simulink model "iff_sim"  (R2019b)
settings: Solver=VariableStepAuto  StartTime=0.0  StopTime=T  FixedStep=0.001  MaxStep=0.001  RelTol=1e-3
values from neighbouring files (symbols this model uses):
  bsc = 17    [model.mat]    (also in model_data.m)
  d_r = [0.01 0.01 0.01 0.01 0.01 0.01]    [model.mat]    (also in model_data.m = 0.01*ones(6,1))
  Fi_b_z = [0 2.09439510239 4.18879020479 1.0471975512 3.14159265359 5.23598775598]    [model.mat]    (also in model_data.m = [0;2/3;4/3;1/3;3/3;5/3]*pi)
  Fp = 148    [model.mat]    (also in model_data.m)
  ka = 11860000    [model.mat]    (also in model_data.m)
  Kd = 0    [ctc_data.m]
  Ki = 0    [ctc_data.m]
  Kp = 300    [ctc_data.m]
  ksc = 179000    [model.mat]    (also in model_data.m)
  l_r = [0.36 0.36 0.36 0.36 0.36 0.36]    [model.mat]    (also in model_data.m = 0.36*ones(6,1))
  la00 = 0.061    [model.mat]    (also in model_data.m)
  O_lb = [0 0 0 0 0 0]    [model.mat]    (also in model_data.m = [0;0;0;0;0;0])
  q_d = out_ik.q'    [ik_run.m]
  qt_d = out_ik.qt'    [ik_run.m]
  qtt_d = out_ik.qtt'    [ik_run.m]
  RMSforce = 35    [model.mat]
  s = out_ctc.s    [ctc_run.m]
  s_0 = s_d(:,:,1)    [ctc_run.m]    (also in iff_run.m)
  T = 1.5    [ctc_data.m]
  t_d = out_ik.t'    [ik_run.m]
  t_dist = 0.1    [model.mat]
  ts_noise = 1.6e-05    [model.mat]    (also in model_data.m)
  v_0 = v_d(:,:,1)    [ctc_run.m]    (also in iff_run.m)
  w_lb = 0.195    [model.mat]    (also in model_data.m)
  W_lb = 0.205    [model.mat]    (also in model_data.m)
  w_ub = 0.195    [model.mat]    (also in model_data.m)
  W_ub = 0.205    [model.mat]    (also in model_data.m)
undefined symbols (not defined in the file or in its folder): X, Y, Z
libraries: nesl_utility x282, sm_lib x208, dspindex x30, simulink x12, powerlib_meascontrol x1
(part 13 of 14)

== system iff_sim/High-authority control/CTC/computed torque control/desired cable vectors// lengths/cable 8 ==
  Cylindrical Joint : sm_lib/Joints/Cylindrical Joint  JointMode=Normal  SenseConstraintForce=off  SenseConstraintForceX=off  SenseConstraintForceY=off  SenseConstraintForceZ=off  SenseConstraintTorque=off  SenseConstraintTorqueX=off  SenseConstraintTorqueY=off  SenseConstraintTorqueZ=off  SenseTotalForce=off  SenseTotalForceX=off  SenseTotalForceY=off  SenseTotalForceZ=off  SenseTotalTorque=off  SenseTotalTorqueX=off  SenseTotalTorqueY=off  SenseTotalTorqueZ=off  CompositeWrenchDir=FollowerOnBase  CompositeWrenchFrame=BaseFrame  PzEquilibriumPosition=0  PzEquilibriumPositionUnits=m  PzSpringStiffness=0  PzSpringStiffnessUnits=N/m  PzDampingCoefficient=0  PzDampingCoefficientUnits=N/(m/s)  PzTorqueActuationMode=ComputedTorque  PzMotionActuationMode=ComputedMotion  PzSensePosition=on  PzSenseVelocity=off  PzSenseAcceleration=off  PzSenseTorqueForce=on  PzSenseLowerLimitTorqueForce=off  PzSenseUpperLimitTorqueForce=off  PzLowerLimitSpecify=off  PzLowerLimitBound=-1  PzLowerLimitBoundUnits=m  PzLowerLimitStiffness=1e6  PzLowerLimitStiffnessUnits=N/m  PzLowerLimitDamping=1e3  PzLowerLimitDampingUnits=N/(m/s)  PzLowerLimitTransitionRegionWidth=1e-4  PzLowerLimitTransitionRegionWidthUnits=m  PzUpperLimitSpecify=off  PzUpperLimitBound=1  PzUpperLimitBoundUnits=m  PzUpperLimitStiffness=1e6  PzUpperLimitStiffnessUnits=N/m  PzUpperLimitDamping=1e3  PzUpperLimitDampingUnits=N/(m/s)  PzUpperLimitTransitionRegionWidth=1e-4  PzUpperLimitTransitionRegionWidthUnits=m  PzPositionTargetSpecify=on  PzPositionTargetPriority=Low  PzPositionTargetValue=1  PzPositionTargetValueUnits=m  PzVelocityTargetSpecify=off  PzVelocityTargetPriority=High  PzVelocityTargetValue=0  PzVelocityTargetValueUnits=m/s  RzEquilibriumPosition=0  RzEquilibriumPositionUnits=deg  RzSpringStiffness=0  RzSpringStiffnessUnits=N*m/deg  RzDampingCoefficient=0  RzDampingCoefficientUnits=N*m/(deg/s)  RzTorqueActuationMode=NoTorque  RzMotionActuationMode=ComputedMotion  RzSensePosition=off  RzSenseVelocity=off  RzSenseAcceleration=off  RzSenseTorqueForce=off  RzSenseLowerLimitTorqueForce=off  RzSenseUpperLimitTorqueForce=off  RzLowerLimitSpecify=off  RzLowerLimitBound=-90  RzLowerLimitBoundUnits=deg  RzLowerLimitStiffness=1e4  RzLowerLimitStiffnessUnits=N*m/deg  RzLowerLimitDamping=10  RzLowerLimitDampingUnits=N*m/(deg/s)  RzLowerLimitTransitionRegionWidth=0.1  RzLowerLimitTransitionRegionWidthUnits=deg  RzUpperLimitSpecify=off  RzUpperLimitBound=90  RzUpperLimitBoundUnits=deg  RzUpperLimitStiffness=1e4  RzUpperLimitStiffnessUnits=N*m/deg  RzUpperLimitDamping=10  RzUpperLimitDampingUnits=N*m/(deg/s)  RzUpperLimitTransitionRegionWidth=0.1  RzUpperLimitTransitionRegionWidthUnits=deg  RzPositionTargetSpecify=off  RzPositionTargetPriority=High  RzPositionTargetValue=0  RzPositionTargetValueUnits=deg  RzVelocityTargetSpecify=off  RzVelocityTargetPriority=High  RzVelocityTargetValue=0  RzVelocityTargetValueUnits=deg/s
  PS-Simulink Converter : nesl_utility/PS-Simulink Converter  PhysicalDomain=network_engine_domain  SubClassName=ps_output  LeftPortType=input  RightPortType=output  PseudoPeriodic=off  Frequencies=[]  Unit=m  AffineConversion=off
  PS-Simulink Converter1 : nesl_utility/PS-Simulink Converter  PhysicalDomain=network_engine_domain  SubClassName=ps_output  LeftPortType=input  RightPortType=output  PseudoPeriodic=off  Frequencies=[]  Unit=N  AffineConversion=off
  Universal Joint : sm_lib/Joints/Universal Joint  JointMode=Normal  SenseConstraintForce=off  SenseConstraintForceX=off  SenseConstraintForceY=off  SenseConstraintForceZ=off  SenseConstraintTorque=off  SenseConstraintTorqueX=off  SenseConstraintTorqueY=off  SenseConstraintTorqueZ=off  SenseTotalForce=off  SenseTotalForceX=off  SenseTotalForceY=off  SenseTotalForceZ=off  SenseTotalTorque=off  SenseTotalTorqueX=off  SenseTotalTorqueY=off  SenseTotalTorqueZ=off  CompositeWrenchDir=FollowerOnBase  CompositeWrenchFrame=BaseFrame  RxEquilibriumPosition=0  RxEquilibriumPositionUnits=deg  RxSpringStiffness=0  RxSpringStiffnessUnits=N*m/deg  RxDampingCoefficient=0  RxDampingCoefficientUnits=N*m/(deg/s)  RxTorqueActuationMode=NoTorque  RxMotionActuationMode=ComputedMotion  RxSensePosition=off  RxSenseVelocity=off  RxSenseAcceleration=off  RxSenseTorqueForce=off  RxSenseLowerLimitTorqueForce=off  RxSenseUpperLimitTorqueForce=off  RxLowerLimitSpecify=off  RxLowerLimitBound=-90  RxLowerLimitBoundUnits=deg  RxLowerLimitStiffness=1e4  RxLowerLimitStiffnessUnits=N*m/deg  RxLowerLimitDamping=10  RxLowerLimitDampingUnits=N*m/(deg/s)  RxLowerLimitTransitionRegionWidth=0.1  RxLowerLimitTransitionRegionWidthUnits=deg  RxUpperLimitSpecify=off  RxUpperLimitBound=90  RxUpperLimitBoundUnits=deg  RxUpperLimitStiffness=1e4  RxUpperLimitStiffnessUnits=N*m/deg  RxUpperLimitDamping=10  RxUpperLimitDampingUnits=N*m/(deg/s)  RxUpperLimitTransitionRegionWidth=0.1  RxUpperLimitTransitionRegionWidthUnits=deg  RxPositionTargetSpecify=off  RxPositionTargetPriority=High  RxPositionTargetValue=0  RxPositionTargetValueUnits=deg  RxVelocityTargetSpecify=off  RxVelocityTargetPriority=High  RxVelocityTargetValue=0  RxVelocityTargetValueUnits=deg/s  RyEquilibriumPosition=0  RyEquilibriumPositionUnits=deg  RySpringStiffness=0  RySpringStiffnessUnits=N*m/deg  RyDampingCoefficient=0  RyDampingCoefficientUnits=N*m/(deg/s)  RyTorqueActuationMode=NoTorque  RyMotionActuationMode=ComputedMotion  RySensePosition=off  RySenseVelocity=off  RySenseAcceleration=off  RySenseTorqueForce=off  RySenseLowerLimitTorqueForce=off  RySenseUpperLimitTorqueForce=off  RyLowerLimitSpecify=off  RyLowerLimitBound=-90  RyLowerLimitBoundUnits=deg  RyLowerLimitStiffness=1e4  RyLowerLimitStiffnessUnits=N*m/deg  RyLowerLimitDamping=10  RyLowerLimitDampingUnits=N*m/(deg/s)  RyLowerLimitTransitionRegionWidth=0.1  RyLowerLimitTransitionRegionWidthUnits=deg  RyUpperLimitSpecify=off  RyUpperLimitBound=90  RyUpperLimitBoundUnits=deg  RyUpperLimitStiffness=1e4  RyUpperLimitStiffnessUnits=N*m/deg  RyUpperLimitDamping=10  RyUpperLimitDampingUnits=N*m/(deg/s)  RyUpperLimitTransitionRegionWidth=0.1  RyUpperLimitTransitionRegionWidthUnits=deg  RyPositionTargetSpecify=off  RyPositionTargetPriority=High  RyPositionTargetValue=0  RyPositionTargetValueUnits=deg  RyVelocityTargetSpecify=off  RyVelocityTargetPriority=High  RyVelocityTargetValue=0  RyVelocityTargetValueUnits=deg/s
      settings: SourceProductName=Simscape Multibody
  Universal Joint1 : sm_lib/Joints/Universal Joint  JointMode=Normal  SenseConstraintForce=off  SenseConstraintForceX=off  SenseConstraintForceY=off  SenseConstraintForceZ=off  SenseConstraintTorque=off  SenseConstraintTorqueX=off  SenseConstraintTorqueY=off  SenseConstraintTorqueZ=off  SenseTotalForce=off  SenseTotalForceX=off  SenseTotalForceY=off  SenseTotalForceZ=off  SenseTotalTorque=off  SenseTotalTorqueX=off  SenseTotalTorqueY=off  SenseTotalTorqueZ=off  CompositeWrenchDir=FollowerOnBase  CompositeWrenchFrame=BaseFrame  RxEquilibriumPosition=0  RxEquilibriumPositionUnits=deg  RxSpringStiffness=0  RxSpringStiffnessUnits=N*m/deg  RxDampingCoefficient=0  RxDampingCoefficientUnits=N*m/(deg/s)  RxTorqueActuationMode=NoTorque  RxMotionActuationMode=ComputedMotion  RxSensePosition=off  RxSenseVelocity=off  RxSenseAcceleration=off  RxSenseTorqueForce=off  RxSenseLowerLimitTorqueForce=off  RxSenseUpperLimitTorqueForce=off  RxLowerLimitSpecify=off  RxLowerLimitBound=-90  RxLowerLimitBoundUnits=deg  RxLowerLimitStiffness=1e4  RxLowerLimitStiffnessUnits=N*m/deg  RxLowerLimitDamping=10  RxLowerLimitDampingUnits=N*m/(deg/s)  RxLowerLimitTransitionRegionWidth=0.1  RxLowerLimitTransitionRegionWidthUnits=deg  RxUpperLimitSpecify=off  RxUpperLimitBound=90  RxUpperLimitBoundUnits=deg  RxUpperLimitStiffness=1e4  RxUpperLimitStiffnessUnits=N*m/deg  RxUpperLimitDamping=10  RxUpperLimitDampingUnits=N*m/(deg/s)  RxUpperLimitTransitionRegionWidth=0.1  RxUpperLimitTransitionRegionWidthUnits=deg  RxPositionTargetSpecify=off  RxPositionTargetPriority=High  RxPositionTargetValue=0  RxPositionTargetValueUnits=deg  RxVelocityTargetSpecify=off  RxVelocityTargetPriority=High  RxVelocityTargetValue=0  RxVelocityTargetValueUnits=deg/s  RyEquilibriumPosition=0  RyEquilibriumPositionUnits=deg  RySpringStiffness=0  RySpringStiffnessUnits=N*m/deg  RyDampingCoefficient=0  RyDampingCoefficientUnits=N*m/(deg/s)  RyTorqueActuationMode=NoTorque  RyMotionActuationMode=ComputedMotion  RySensePosition=off  RySenseVelocity=off  RySenseAcceleration=off  RySenseTorqueForce=off  RySenseLowerLimitTorqueForce=off  RySenseUpperLimitTorqueForce=off  RyLowerLimitSpecify=off  RyLowerLimitBound=-90  RyLowerLimitBoundUnits=deg  RyLowerLimitStiffness=1e4  RyLowerLimitStiffnessUnits=N*m/deg  RyLowerLimitDamping=10  RyLowerLimitDampingUnits=N*m/(deg/s)  RyLowerLimitTransitionRegionWidth=0.1  RyLowerLimitTransitionRegionWidthUnits=deg  RyUpperLimitSpecify=off  RyUpperLimitBound=90  RyUpperLimitBoundUnits=deg  RyUpperLimitStiffness=1e4  RyUpperLimitStiffnessUnits=N*m/deg  RyUpperLimitDamping=10  RyUpperLimitDampingUnits=N*m/(deg/s)  RyUpperLimitTransitionRegionWidth=0.1  RyUpperLimitTransitionRegionWidthUnits=deg  RyPositionTargetSpecify=off  RyPositionTargetPriority=High  RyPositionTargetValue=0  RyPositionTargetValueUnits=deg  RyVelocityTargetSpecify=off  RyVelocityTargetPriority=High  RyVelocityTargetValue=0  RyVelocityTargetValueUnits=deg/s
      settings: SourceProductName=Simscape Multibody
  cable force and length : MATLAB Function  TreatAsAtomicUnit=on
  K_c : PMIOPort  Side=Left
  L_c : PMIOPort  Port=2  Side=Right
  F_c : Outport
  l_c : Outport  Port=2
  wires:
  PS-Simulink Converter/1 -> cable force and length/1(pz)
  PS-Simulink Converter1/1 -> cable force and length/2(fz)
  cable force and length/1(F_c) -> F_c/1
  cable force and length/2(l_c) -> l_c/1
  connections:
  Universal Joint/LConn1 -- K_c/RConn1
  Cylindrical Joint/LConn1 -- Universal Joint/RConn1
  L_c/RConn1 -- Universal Joint1/RConn1
  Universal Joint1/LConn1 -- Cylindrical Joint/RConn1
  PS-Simulink Converter/LConn1 -- Cylindrical Joint/RConn2
  PS-Simulink Converter1/LConn1 -- Cylindrical Joint/RConn3

== system iff_sim/High-authority control/CTC/computed torque control/desired cable vectors// lengths/cable 9 ==
  Cylindrical Joint : sm_lib/Joints/Cylindrical Joint  JointMode=Normal  SenseConstraintForce=off  SenseConstraintForceX=off  SenseConstraintForceY=off  SenseConstraintForceZ=off  SenseConstraintTorque=off  SenseConstraintTorqueX=off  SenseConstraintTorqueY=off  SenseConstraintTorqueZ=off  SenseTotalForce=off  SenseTotalForceX=off  SenseTotalForceY=off  SenseTotalForceZ=off  SenseTotalTorque=off  SenseTotalTorqueX=off  SenseTotalTorqueY=off  SenseTotalTorqueZ=off  CompositeWrenchDir=FollowerOnBase  CompositeWrenchFrame=BaseFrame  PzEquilibriumPosition=0  PzEquilibriumPositionUnits=m  PzSpringStiffness=0  PzSpringStiffnessUnits=N/m  PzDampingCoefficient=0  PzDampingCoefficientUnits=N/(m/s)  PzTorqueActuationMode=ComputedTorque  PzMotionActuationMode=ComputedMotion  PzSensePosition=on  PzSenseVelocity=off  PzSenseAcceleration=off  PzSenseTorqueForce=on  PzSenseLowerLimitTorqueForce=off  PzSenseUpperLimitTorqueForce=off  PzLowerLimitSpecify=off  PzLowerLimitBound=-1  PzLowerLimitBoundUnits=m  PzLowerLimitStiffness=1e6  PzLowerLimitStiffnessUnits=N/m  PzLowerLimitDamping=1e3  PzLowerLimitDampingUnits=N/(m/s)  PzLowerLimitTransitionRegionWidth=1e-4  PzLowerLimitTransitionRegionWidthUnits=m  PzUpperLimitSpecify=off  PzUpperLimitBound=1  PzUpperLimitBoundUnits=m  PzUpperLimitStiffness=1e6  PzUpperLimitStiffnessUnits=N/m  PzUpperLimitDamping=1e3  PzUpperLimitDampingUnits=N/(m/s)  PzUpperLimitTransitionRegionWidth=1e-4  PzUpperLimitTransitionRegionWidthUnits=m  PzPositionTargetSpecify=on  PzPositionTargetPriority=Low  PzPositionTargetValue=1  PzPositionTargetValueUnits=m  PzVelocityTargetSpecify=off  PzVelocityTargetPriority=High  PzVelocityTargetValue=0  PzVelocityTargetValueUnits=m/s  RzEquilibriumPosition=0  RzEquilibriumPositionUnits=deg  RzSpringStiffness=0  RzSpringStiffnessUnits=N*m/deg  RzDampingCoefficient=0  RzDampingCoefficientUnits=N*m/(deg/s)  RzTorqueActuationMode=NoTorque  RzMotionActuationMode=ComputedMotion  RzSensePosition=off  RzSenseVelocity=off  RzSenseAcceleration=off  RzSenseTorqueForce=off  RzSenseLowerLimitTorqueForce=off  RzSenseUpperLimitTorqueForce=off  RzLowerLimitSpecify=off  RzLowerLimitBound=-90  RzLowerLimitBoundUnits=deg  RzLowerLimitStiffness=1e4  RzLowerLimitStiffnessUnits=N*m/deg  RzLowerLimitDamping=10  RzLowerLimitDampingUnits=N*m/(deg/s)  RzLowerLimitTransitionRegionWidth=0.1  RzLowerLimitTransitionRegionWidthUnits=deg  RzUpperLimitSpecify=off  RzUpperLimitBound=90  RzUpperLimitBoundUnits=deg  RzUpperLimitStiffness=1e4  RzUpperLimitStiffnessUnits=N*m/deg  RzUpperLimitDamping=10  RzUpperLimitDampingUnits=N*m/(deg/s)  RzUpperLimitTransitionRegionWidth=0.1  RzUpperLimitTransitionRegionWidthUnits=deg  RzPositionTargetSpecify=off  RzPositionTargetPriority=High  RzPositionTargetValue=0  RzPositionTargetValueUnits=deg  RzVelocityTargetSpecify=off  RzVelocityTargetPriority=High  RzVelocityTargetValue=0  RzVelocityTargetValueUnits=deg/s
  PS-Simulink Converter : nesl_utility/PS-Simulink Converter  PhysicalDomain=network_engine_domain  SubClassName=ps_output  LeftPortType=input  RightPortType=output  PseudoPeriodic=off  Frequencies=[]  Unit=m  AffineConversion=off
  PS-Simulink Converter1 : nesl_utility/PS-Simulink Converter  PhysicalDomain=network_engine_domain  SubClassName=ps_output  LeftPortType=input  RightPortType=output  PseudoPeriodic=off  Frequencies=[]  Unit=N  AffineConversion=off
  Universal Joint : sm_lib/Joints/Universal Joint  JointMode=Normal  SenseConstraintForce=off  SenseConstraintForceX=off  SenseConstraintForceY=off  SenseConstraintForceZ=off  SenseConstraintTorque=off  SenseConstraintTorqueX=off  SenseConstraintTorqueY=off  SenseConstraintTorqueZ=off  SenseTotalForce=off  SenseTotalForceX=off  SenseTotalForceY=off  SenseTotalForceZ=off  SenseTotalTorque=off  SenseTotalTorqueX=off  SenseTotalTorqueY=off  SenseTotalTorqueZ=off  CompositeWrenchDir=FollowerOnBase  CompositeWrenchFrame=BaseFrame  RxEquilibriumPosition=0  RxEquilibriumPositionUnits=deg  RxSpringStiffness=0  RxSpringStiffnessUnits=N*m/deg  RxDampingCoefficient=0  RxDampingCoefficientUnits=N*m/(deg/s)  RxTorqueActuationMode=NoTorque  RxMotionActuationMode=ComputedMotion  RxSensePosition=off  RxSenseVelocity=off  RxSenseAcceleration=off  RxSenseTorqueForce=off  RxSenseLowerLimitTorqueForce=off  RxSenseUpperLimitTorqueForce=off  RxLowerLimitSpecify=off  RxLowerLimitBound=-90  RxLowerLimitBoundUnits=deg  RxLowerLimitStiffness=1e4  RxLowerLimitStiffnessUnits=N*m/deg  RxLowerLimitDamping=10  RxLowerLimitDampingUnits=N*m/(deg/s)  RxLowerLimitTransitionRegionWidth=0.1  RxLowerLimitTransitionRegionWidthUnits=deg  RxUpperLimitSpecify=off  RxUpperLimitBound=90  RxUpperLimitBoundUnits=deg  RxUpperLimitStiffness=1e4  RxUpperLimitStiffnessUnits=N*m/deg  RxUpperLimitDamping=10  RxUpperLimitDampingUnits=N*m/(deg/s)  RxUpperLimitTransitionRegionWidth=0.1  RxUpperLimitTransitionRegionWidthUnits=deg  RxPositionTargetSpecify=off  RxPositionTargetPriority=High  RxPositionTargetValue=0  RxPositionTargetValueUnits=deg  RxVelocityTargetSpecify=off  RxVelocityTargetPriority=High  RxVelocityTargetValue=0  RxVelocityTargetValueUnits=deg/s  RyEquilibriumPosition=0  RyEquilibriumPositionUnits=deg  RySpringStiffness=0  RySpringStiffnessUnits=N*m/deg  RyDampingCoefficient=0  RyDampingCoefficientUnits=N*m/(deg/s)  RyTorqueActuationMode=NoTorque  RyMotionActuationMode=ComputedMotion  RySensePosition=off  RySenseVelocity=off  RySenseAcceleration=off  RySenseTorqueForce=off  RySenseLowerLimitTorqueForce=off  RySenseUpperLimitTorqueForce=off  RyLowerLimitSpecify=off  RyLowerLimitBound=-90  RyLowerLimitBoundUnits=deg  RyLowerLimitStiffness=1e4  RyLowerLimitStiffnessUnits=N*m/deg  RyLowerLimitDamping=10  RyLowerLimitDampingUnits=N*m/(deg/s)  RyLowerLimitTransitionRegionWidth=0.1  RyLowerLimitTransitionRegionWidthUnits=deg  RyUpperLimitSpecify=off  RyUpperLimitBound=90  RyUpperLimitBoundUnits=deg  RyUpperLimitStiffness=1e4  RyUpperLimitStiffnessUnits=N*m/deg  RyUpperLimitDamping=10  RyUpperLimitDampingUnits=N*m/(deg/s)  RyUpperLimitTransitionRegionWidth=0.1  RyUpperLimitTransitionRegionWidthUnits=deg  RyPositionTargetSpecify=off  RyPositionTargetPriority=High  RyPositionTargetValue=0  RyPositionTargetValueUnits=deg  RyVelocityTargetSpecify=off  RyVelocityTargetPriority=High  RyVelocityTargetValue=0  RyVelocityTargetValueUnits=deg/s
      settings: SourceProductName=Simscape Multibody
  Universal Joint1 : sm_lib/Joints/Universal Joint  JointMode=Normal  SenseConstraintForce=off  SenseConstraintForceX=off  SenseConstraintForceY=off  SenseConstraintForceZ=off  SenseConstraintTorque=off  SenseConstraintTorqueX=off  SenseConstraintTorqueY=off  SenseConstraintTorqueZ=off  SenseTotalForce=off  SenseTotalForceX=off  SenseTotalForceY=off  SenseTotalForceZ=off  SenseTotalTorque=off  SenseTotalTorqueX=off  SenseTotalTorqueY=off  SenseTotalTorqueZ=off  CompositeWrenchDir=FollowerOnBase  CompositeWrenchFrame=BaseFrame  RxEquilibriumPosition=0  RxEquilibriumPositionUnits=deg  RxSpringStiffness=0  RxSpringStiffnessUnits=N*m/deg  RxDampingCoefficient=0  RxDampingCoefficientUnits=N*m/(deg/s)  RxTorqueActuationMode=NoTorque  RxMotionActuationMode=ComputedMotion  RxSensePosition=off  RxSenseVelocity=off  RxSenseAcceleration=off  RxSenseTorqueForce=off  RxSenseLowerLimitTorqueForce=off  RxSenseUpperLimitTorqueForce=off  RxLowerLimitSpecify=off  RxLowerLimitBound=-90  RxLowerLimitBoundUnits=deg  RxLowerLimitStiffness=1e4  RxLowerLimitStiffnessUnits=N*m/deg  RxLowerLimitDamping=10  RxLowerLimitDampingUnits=N*m/(deg/s)  RxLowerLimitTransitionRegionWidth=0.1  RxLowerLimitTransitionRegionWidthUnits=deg  RxUpperLimitSpecify=off  RxUpperLimitBound=90  RxUpperLimitBoundUnits=deg  RxUpperLimitStiffness=1e4  RxUpperLimitStiffnessUnits=N*m/deg  RxUpperLimitDamping=10  RxUpperLimitDampingUnits=N*m/(deg/s)  RxUpperLimitTransitionRegionWidth=0.1  RxUpperLimitTransitionRegionWidthUnits=deg  RxPositionTargetSpecify=off  RxPositionTargetPriority=High  RxPositionTargetValue=0  RxPositionTargetValueUnits=deg  RxVelocityTargetSpecify=off  RxVelocityTargetPriority=High  RxVelocityTargetValue=0  RxVelocityTargetValueUnits=deg/s  RyEquilibriumPosition=0  RyEquilibriumPositionUnits=deg  RySpringStiffness=0  RySpringStiffnessUnits=N*m/deg  RyDampingCoefficient=0  RyDampingCoefficientUnits=N*m/(deg/s)  RyTorqueActuationMode=NoTorque  RyMotionActuationMode=ComputedMotion  RySensePosition=off  RySenseVelocity=off  RySenseAcceleration=off  RySenseTorqueForce=off  RySenseLowerLimitTorqueForce=off  RySenseUpperLimitTorqueForce=off  RyLowerLimitSpecify=off  RyLowerLimitBound=-90  RyLowerLimitBoundUnits=deg  RyLowerLimitStiffness=1e4  RyLowerLimitStiffnessUnits=N*m/deg  RyLowerLimitDamping=10  RyLowerLimitDampingUnits=N*m/(deg/s)  RyLowerLimitTransitionRegionWidth=0.1  RyLowerLimitTransitionRegionWidthUnits=deg  RyUpperLimitSpecify=off  RyUpperLimitBound=90  RyUpperLimitBoundUnits=deg  RyUpperLimitStiffness=1e4  RyUpperLimitStiffnessUnits=N*m/deg  RyUpperLimitDamping=10  RyUpperLimitDampingUnits=N*m/(deg/s)  RyUpperLimitTransitionRegionWidth=0.1  RyUpperLimitTransitionRegionWidthUnits=deg  RyPositionTargetSpecify=off  RyPositionTargetPriority=High  RyPositionTargetValue=0  RyPositionTargetValueUnits=deg  RyVelocityTargetSpecify=off  RyVelocityTargetPriority=High  RyVelocityTargetValue=0  RyVelocityTargetValueUnits=deg/s
      settings: SourceProductName=Simscape Multibody
  cable force and length : MATLAB Function  TreatAsAtomicUnit=on
  K_c : PMIOPort  Side=Left
  L_c : PMIOPort  Port=2  Side=Right
  F_c : Outport
  l_c : Outport  Port=2
  wires:
  PS-Simulink Converter/1 -> cable force and length/1(pz)
  PS-Simulink Converter1/1 -> cable force and length/2(fz)
  cable force and length/1(F_c) -> F_c/1
  cable force and length/2(l_c) -> l_c/1
  connections:
  Universal Joint/LConn1 -- K_c/RConn1
  Cylindrical Joint/LConn1 -- Universal Joint/RConn1
  L_c/RConn1 -- Universal Joint1/RConn1
  Universal Joint1/LConn1 -- Cylindrical Joint/RConn1
  PS-Simulink Converter/LConn1 -- Cylindrical Joint/RConn2
  PS-Simulink Converter1/LConn1 -- Cylindrical Joint/RConn3

== system iff_sim/High-authority control/CTC/inverse kinematics/t -> q_d/rod 1 ==
  t : Inport
  Mux : Mux  Inputs=2
  Q_r,d,x : Lookup_n-D  NumberOfTableDimensions=1  BreakpointsForDimension1=t_d(1,:)  BreakpointsForDimension2=t_d(1,:)  Table=Q_d((r-1)*2+1,:)  InternalRulePriority=Speed  RndMeth=Simplest  InputSameDT=on
  Q_r,d,y : Lookup_n-D  NumberOfTableDimensions=1  BreakpointsForDimension1=t_d(1,:)  BreakpointsForDimension2=t_d(1,:)  Table=Q_d((r-1)*2+2,:)  InternalRulePriority=Speed  RndMeth=Simplest  InputSameDT=on
  Q_r,d : Outport
  wires:
  t/1 -> Q_r,d,y/1, Q_r,d,x/1
  Q_r,d,y/1 -> Mux/2
  Q_r,d,x/1 -> Mux/1
  Mux/1 -> Q_r,d/1

== system iff_sim/High-authority control/CTC/inverse kinematics/t -> q_d/rod 2 ==
  t : Inport
  Mux : Mux  Inputs=2
  Q_r,d,x : Lookup_n-D  NumberOfTableDimensions=1  BreakpointsForDimension1=t_d(1,:)  BreakpointsForDimension2=t_d(1,:)  Table=Q_d((r-1)*2+1,:)  InternalRulePriority=Speed  RndMeth=Simplest  InputSameDT=on
  Q_r,d,y : Lookup_n-D  NumberOfTableDimensions=1  BreakpointsForDimension1=t_d(1,:)  BreakpointsForDimension2=t_d(1,:)  Table=Q_d((r-1)*2+2,:)  InternalRulePriority=Speed  RndMeth=Simplest  InputSameDT=on
  Q_r,d : Outport
  wires:
  t/1 -> Q_r,d,y/1, Q_r,d,x/1
  Q_r,d,y/1 -> Mux/2
  Q_r,d,x/1 -> Mux/1
  Mux/1 -> Q_r,d/1

== system iff_sim/High-authority control/CTC/inverse kinematics/t -> q_d/rod 3 ==
  t : Inport
  Mux : Mux  Inputs=2
  Q_r,d,x : Lookup_n-D  NumberOfTableDimensions=1  BreakpointsForDimension1=t_d(1,:)  BreakpointsForDimension2=t_d(1,:)  Table=Q_d((r-1)*2+1,:)  InternalRulePriority=Speed  RndMeth=Simplest  InputSameDT=on
  Q_r,d,y : Lookup_n-D  NumberOfTableDimensions=1  BreakpointsForDimension1=t_d(1,:)  BreakpointsForDimension2=t_d(1,:)  Table=Q_d((r-1)*2+2,:)  InternalRulePriority=Speed  RndMeth=Simplest  InputSameDT=on
  Q_r,d : Outport
  wires:
  t/1 -> Q_r,d,y/1, Q_r,d,x/1
  Q_r,d,y/1 -> Mux/2
  Q_r,d,x/1 -> Mux/1
  Mux/1 -> Q_r,d/1

== system iff_sim/High-authority control/CTC/inverse kinematics/t -> q_d/rod 4 ==
  t : Inport
  Mux : Mux  Inputs=2
  Q_r,d,x : Lookup_n-D  NumberOfTableDimensions=1  BreakpointsForDimension1=t_d(1,:)  BreakpointsForDimension2=t_d(1,:)  Table=Q_d((r-1)*2+1,:)  InternalRulePriority=Speed  RndMeth=Simplest  InputSameDT=on
  Q_r,d,y : Lookup_n-D  NumberOfTableDimensions=1  BreakpointsForDimension1=t_d(1,:)  BreakpointsForDimension2=t_d(1,:)  Table=Q_d((r-1)*2+2,:)  InternalRulePriority=Speed  RndMeth=Simplest  InputSameDT=on
  Q_r,d : Outport
  wires:
  t/1 -> Q_r,d,y/1, Q_r,d,x/1
  Q_r,d,y/1 -> Mux/2
  Q_r,d,x/1 -> Mux/1
  Mux/1 -> Q_r,d/1

== system iff_sim/High-authority control/CTC/inverse kinematics/t -> q_d/rod 5 ==
  t : Inport
  Mux : Mux  Inputs=2
  Q_r,d,x : Lookup_n-D  NumberOfTableDimensions=1  BreakpointsForDimension1=t_d(1,:)  BreakpointsForDimension2=t_d(1,:)  Table=Q_d((r-1)*2+1,:)  InternalRulePriority=Speed  RndMeth=Simplest  InputSameDT=on
  Q_r,d,y : Lookup_n-D  NumberOfTableDimensions=1  BreakpointsForDimension1=t_d(1,:)  BreakpointsForDimension2=t_d(1,:)  Table=Q_d((r-1)*2+2,:)  InternalRulePriority=Speed  RndMeth=Simplest  InputSameDT=on
  Q_r,d : Outport
  wires:
  t/1 -> Q_r,d,y/1, Q_r,d,x/1
  Q_r,d,y/1 -> Mux/2
  Q_r,d,x/1 -> Mux/1
  Mux/1 -> Q_r,d/1

== system iff_sim/High-authority control/CTC/inverse kinematics/t -> q_d/rod 6 ==
  t : Inport
  Mux : Mux  Inputs=2
  Q_r,d,x : Lookup_n-D  NumberOfTableDimensions=1  BreakpointsForDimension1=t_d(1,:)  BreakpointsForDimension2=t_d(1,:)  Table=Q_d((r-1)*2+1,:)  InternalRulePriority=Speed  RndMeth=Simplest  InputSameDT=on
  Q_r,d,y : Lookup_n-D  NumberOfTableDimensions=1  BreakpointsForDimension1=t_d(1,:)  BreakpointsForDimension2=t_d(1,:)  Table=Q_d((r-1)*2+2,:)  InternalRulePriority=Speed  RndMeth=Simplest  InputSameDT=on
  Q_r,d : Outport
  wires:
  t/1 -> Q_r,d,y/1, Q_r,d,x/1
  Q_r,d,y/1 -> Mux/2
  Q_r,d,x/1 -> Mux/1
  Mux/1 -> Q_r,d/1

== system iff_sim/High-authority control/CTC/inverse kinematics/t -> q_d/upper base ==
  t : Inport
  Mux : Mux  Inputs=6
  Q_ub,d,phi_x : Lookup_n-D  NumberOfTableDimensions=1  BreakpointsForDimension1=t_d(1,:)  BreakpointsForDimension2=t_d(1,:)  Table=Q_d(16,:)  InternalRulePriority=Speed  RndMeth=Simplest  InputSameDT=on
  Q_ub,d,phi_y : Lookup_n-D  NumberOfTableDimensions=1  BreakpointsForDimension1=t_d(1,:)  BreakpointsForDimension2=t_d(1,:)  Table=Q_d(17,:)  InternalRulePriority=Speed  RndMeth=Simplest  InputSameDT=on
  Q_ub,d,phi_z : Lookup_n-D  NumberOfTableDimensions=1  BreakpointsForDimension1=t_d(1,:)  BreakpointsForDimension2=t_d(1,:)  Table=Q_d(18,:)  InternalRulePriority=Speed  RndMeth=Simplest  InputSameDT=on
  Q_ub,d,x : Lookup_n-D  NumberOfTableDimensions=1  BreakpointsForDimension1=t_d(1,:)  BreakpointsForDimension2=t_d(1,:)  Table=Q_d(13,:)  InternalRulePriority=Speed  RndMeth=Simplest  InputSameDT=on
  Q_ub,d,y : Lookup_n-D  NumberOfTableDimensions=1  BreakpointsForDimension1=t_d(1,:)  BreakpointsForDimension2=t_d(1,:)  Table=Q_d(14,:)  InternalRulePriority=Speed  RndMeth=Simplest  InputSameDT=on
  Q_ub,d,z : Lookup_n-D  NumberOfTableDimensions=1  BreakpointsForDimension1=t_d(1,:)  BreakpointsForDimension2=t_d(1,:)  Table=Q_d(15,:)  InternalRulePriority=Speed  RndMeth=Simplest  InputSameDT=on
  Q_ub,d : Outport
  wires:
  t/1 -> Q_ub,d,y/1, Q_ub,d,z/1, Q_ub,d,phi_x/1, Q_ub,d,phi_y/1, Q_ub,d,phi_z/1, Q_ub,d,x/1
  Q_ub,d,x/1 -> Mux/1
  Q_ub,d,phi_z/1 -> Mux/6
  Q_ub,d,phi_y/1 -> Mux/5
  Q_ub,d,phi_x/1 -> Mux/4
  Q_ub,d,z/1 -> Mux/3
  Q_ub,d,y/1 -> Mux/2
  Mux/1 -> Q_ub,d/1

== system iff_sim/High-authority control/CTC/inverse kinematics/t -> qt_d/rod 1 ==
  t : Inport
  Mux : Mux  Inputs=2
  Q_r,d,x : Lookup_n-D  NumberOfTableDimensions=1  BreakpointsForDimension1=t_d(1,:)  BreakpointsForDimension2=t_d(1,:)  Table=Q_d((r-1)*2+1,:)  InternalRulePriority=Speed  RndMeth=Simplest  InputSameDT=on
  Q_r,d,y : Lookup_n-D  NumberOfTableDimensions=1  BreakpointsForDimension1=t_d(1,:)  BreakpointsForDimension2=t_d(1,:)  Table=Q_d((r-1)*2+2,:)  InternalRulePriority=Speed  RndMeth=Simplest  InputSameDT=on
  Q_r,d : Outport
  wires:
  t/1 -> Q_r,d,y/1, Q_r,d,x/1
  Q_r,d,y/1 -> Mux/2
  Q_r,d,x/1 -> Mux/1
  Mux/1 -> Q_r,d/1

== system iff_sim/High-authority control/CTC/inverse kinematics/t -> qt_d/rod 2 ==
  t : Inport
  Mux : Mux  Inputs=2
  Q_r,d,x : Lookup_n-D  NumberOfTableDimensions=1  BreakpointsForDimension1=t_d(1,:)  BreakpointsForDimension2=t_d(1,:)  Table=Q_d((r-1)*2+1,:)  InternalRulePriority=Speed  RndMeth=Simplest  InputSameDT=on
  Q_r,d,y : Lookup_n-D  NumberOfTableDimensions=1  BreakpointsForDimension1=t_d(1,:)  BreakpointsForDimension2=t_d(1,:)  Table=Q_d((r-1)*2+2,:)  InternalRulePriority=Speed  RndMeth=Simplest  InputSameDT=on
  Q_r,d : Outport
  wires:
  t/1 -> Q_r,d,y/1, Q_r,d,x/1
  Q_r,d,y/1 -> Mux/2
  Q_r,d,x/1 -> Mux/1
  Mux/1 -> Q_r,d/1

== system iff_sim/High-authority control/CTC/inverse kinematics/t -> qt_d/rod 3 ==
  t : Inport
  Mux : Mux  Inputs=2
  Q_r,d,x : Lookup_n-D  NumberOfTableDimensions=1  BreakpointsForDimension1=t_d(1,:)  BreakpointsForDimension2=t_d(1,:)  Table=Q_d((r-1)*2+1,:)  InternalRulePriority=Speed  RndMeth=Simplest  InputSameDT=on
  Q_r,d,y : Lookup_n-D  NumberOfTableDimensions=1  BreakpointsForDimension1=t_d(1,:)  BreakpointsForDimension2=t_d(1,:)  Table=Q_d((r-1)*2+2,:)  InternalRulePriority=Speed  RndMeth=Simplest  InputSameDT=on
  Q_r,d : Outport
  wires:
  t/1 -> Q_r,d,y/1, Q_r,d,x/1
  Q_r,d,y/1 -> Mux/2
  Q_r,d,x/1 -> Mux/1
  Mux/1 -> Q_r,d/1

== system iff_sim/High-authority control/CTC/inverse kinematics/t -> qt_d/rod 4 ==
  t : Inport
  Mux : Mux  Inputs=2
  Q_r,d,x : Lookup_n-D  NumberOfTableDimensions=1  BreakpointsForDimension1=t_d(1,:)  BreakpointsForDimension2=t_d(1,:)  Table=Q_d((r-1)*2+1,:)  InternalRulePriority=Speed  RndMeth=Simplest  InputSameDT=on
  Q_r,d,y : Lookup_n-D  NumberOfTableDimensions=1  BreakpointsForDimension1=t_d(1,:)  BreakpointsForDimension2=t_d(1,:)  Table=Q_d((r-1)*2+2,:)  InternalRulePriority=Speed  RndMeth=Simplest  InputSameDT=on
  Q_r,d : Outport
  wires:
  t/1 -> Q_r,d,y/1, Q_r,d,x/1
  Q_r,d,y/1 -> Mux/2
  Q_r,d,x/1 -> Mux/1
  Mux/1 -> Q_r,d/1

== system iff_sim/High-authority control/CTC/inverse kinematics/t -> qt_d/rod 5 ==
  t : Inport
  Mux : Mux  Inputs=2
  Q_r,d,x : Lookup_n-D  NumberOfTableDimensions=1  BreakpointsForDimension1=t_d(1,:)  BreakpointsForDimension2=t_d(1,:)  Table=Q_d((r-1)*2+1,:)  InternalRulePriority=Speed  RndMeth=Simplest  InputSameDT=on
  Q_r,d,y : Lookup_n-D  NumberOfTableDimensions=1  BreakpointsForDimension1=t_d(1,:)  BreakpointsForDimension2=t_d(1,:)  Table=Q_d((r-1)*2+2,:)  InternalRulePriority=Speed  RndMeth=Simplest  InputSameDT=on
  Q_r,d : Outport
  wires:
  t/1 -> Q_r,d,y/1, Q_r,d,x/1
  Q_r,d,y/1 -> Mux/2
  Q_r,d,x/1 -> Mux/1
  Mux/1 -> Q_r,d/1

== system iff_sim/High-authority control/CTC/inverse kinematics/t -> qt_d/rod 6 ==
  t : Inport
  Mux : Mux  Inputs=2
  Q_r,d,x : Lookup_n-D  NumberOfTableDimensions=1  BreakpointsForDimension1=t_d(1,:)  BreakpointsForDimension2=t_d(1,:)  Table=Q_d((r-1)*2+1,:)  InternalRulePriority=Speed  RndMeth=Simplest  InputSameDT=on
  Q_r,d,y : Lookup_n-D  NumberOfTableDimensions=1  BreakpointsForDimension1=t_d(1,:)  BreakpointsForDimension2=t_d(1,:)  Table=Q_d((r-1)*2+2,:)  InternalRulePriority=Speed  RndMeth=Simplest  InputSameDT=on
  Q_r,d : Outport
  wires:
  t/1 -> Q_r,d,y/1, Q_r,d,x/1
  Q_r,d,y/1 -> Mux/2
  Q_r,d,x/1 -> Mux/1
  Mux/1 -> Q_r,d/1

== system iff_sim/High-authority control/CTC/inverse kinematics/t -> qt_d/upper base ==
  t : Inport
  Mux : Mux  Inputs=6
  Q_ub,d,phi_x : Lookup_n-D  NumberOfTableDimensions=1  BreakpointsForDimension1=t_d(1,:)  BreakpointsForDimension2=t_d(1,:)  Table=Q_d(16,:)  InternalRulePriority=Speed  RndMeth=Simplest  InputSameDT=on
  Q_ub,d,phi_y : Lookup_n-D  NumberOfTableDimensions=1  BreakpointsForDimension1=t_d(1,:)  BreakpointsForDimension2=t_d(1,:)  Table=Q_d(17,:)  InternalRulePriority=Speed  RndMeth=Simplest  InputSameDT=on
  Q_ub,d,phi_z : Lookup_n-D  NumberOfTableDimensions=1  BreakpointsForDimension1=t_d(1,:)  BreakpointsForDimension2=t_d(1,:)  Table=Q_d(18,:)  InternalRulePriority=Speed  RndMeth=Simplest  InputSameDT=on
  Q_ub,d,x : Lookup_n-D  NumberOfTableDimensions=1  BreakpointsForDimension1=t_d(1,:)  BreakpointsForDimension2=t_d(1,:)  Table=Q_d(13,:)  InternalRulePriority=Speed  RndMeth=Simplest  InputSameDT=on
  Q_ub,d,y : Lookup_n-D  NumberOfTableDimensions=1  BreakpointsForDimension1=t_d(1,:)  BreakpointsForDimension2=t_d(1,:)  Table=Q_d(14,:)  InternalRulePriority=Speed  RndMeth=Simplest  InputSameDT=on
  Q_ub,d,z : Lookup_n-D  NumberOfTableDimensions=1  BreakpointsForDimension1=t_d(1,:)  BreakpointsForDimension2=t_d(1,:)  Table=Q_d(15,:)  InternalRulePriority=Speed  RndMeth=Simplest  InputSameDT=on
  Q_ub,d : Outport
  wires:
  t/1 -> Q_ub,d,y/1, Q_ub,d,z/1, Q_ub,d,phi_x/1, Q_ub,d,phi_y/1, Q_ub,d,phi_z/1, Q_ub,d,x/1
  Q_ub,d,x/1 -> Mux/1
  Q_ub,d,phi_z/1 -> Mux/6
  Q_ub,d,phi_y/1 -> Mux/5
  Q_ub,d,phi_x/1 -> Mux/4
  Q_ub,d,z/1 -> Mux/3
  Q_ub,d,y/1 -> Mux/2
  Mux/1 -> Q_ub,d/1

== system iff_sim/High-authority control/CTC/inverse kinematics/t -> qtt_d/rod 1 ==
  t : Inport
  Mux : Mux  Inputs=2
  Q_r,d,x : Lookup_n-D  NumberOfTableDimensions=1  BreakpointsForDimension1=t_d(1,:)  BreakpointsForDimension2=t_d(1,:)  Table=Q_d((r-1)*2+1,:)  InternalRulePriority=Speed  RndMeth=Simplest  InputSameDT=on
  Q_r,d,y : Lookup_n-D  NumberOfTableDimensions=1  BreakpointsForDimension1=t_d(1,:)  BreakpointsForDimension2=t_d(1,:)  Table=Q_d((r-1)*2+2,:)  InternalRulePriority=Speed  RndMeth=Simplest  InputSameDT=on
  Q_r,d : Outport
  wires:
  t/1 -> Q_r,d,y/1, Q_r,d,x/1
  Q_r,d,y/1 -> Mux/2
  Q_r,d,x/1 -> Mux/1
  Mux/1 -> Q_r,d/1

== system iff_sim/High-authority control/CTC/inverse kinematics/t -> qtt_d/rod 2 ==
  t : Inport
  Mux : Mux  Inputs=2
  Q_r,d,x : Lookup_n-D  NumberOfTableDimensions=1  BreakpointsForDimension1=t_d(1,:)  BreakpointsForDimension2=t_d(1,:)  Table=Q_d((r-1)*2+1,:)  InternalRulePriority=Speed  RndMeth=Simplest  InputSameDT=on
  Q_r,d,y : Lookup_n-D  NumberOfTableDimensions=1  BreakpointsForDimension1=t_d(1,:)  BreakpointsForDimension2=t_d(1,:)  Table=Q_d((r-1)*2+2,:)  InternalRulePriority=Speed  RndMeth=Simplest  InputSameDT=on
  Q_r,d : Outport
  wires:
  t/1 -> Q_r,d,y/1, Q_r,d,x/1
  Q_r,d,y/1 -> Mux/2
  Q_r,d,x/1 -> Mux/1
  Mux/1 -> Q_r,d/1

== system iff_sim/High-authority control/CTC/inverse kinematics/t -> qtt_d/rod 3 ==
  t : Inport
  Mux : Mux  Inputs=2
  Q_r,d,x : Lookup_n-D  NumberOfTableDimensions=1  BreakpointsForDimension1=t_d(1,:)  BreakpointsForDimension2=t_d(1,:)  Table=Q_d((r-1)*2+1,:)  InternalRulePriority=Speed  RndMeth=Simplest  InputSameDT=on
  Q_r,d,y : Lookup_n-D  NumberOfTableDimensions=1  BreakpointsForDimension1=t_d(1,:)  BreakpointsForDimension2=t_d(1,:)  Table=Q_d((r-1)*2+2,:)  InternalRulePriority=Speed  RndMeth=Simplest  InputSameDT=on
  Q_r,d : Outport
  wires:
  t/1 -> Q_r,d,y/1, Q_r,d,x/1
  Q_r,d,y/1 -> Mux/2
  Q_r,d,x/1 -> Mux/1
  Mux/1 -> Q_r,d/1

== system iff_sim/High-authority control/CTC/inverse kinematics/t -> qtt_d/rod 4 ==
  t : Inport
  Mux : Mux  Inputs=2
  Q_r,d,x : Lookup_n-D  NumberOfTableDimensions=1  BreakpointsForDimension1=t_d(1,:)  BreakpointsForDimension2=t_d(1,:)  Table=Q_d((r-1)*2+1,:)  InternalRulePriority=Speed  RndMeth=Simplest  InputSameDT=on
  Q_r,d,y : Lookup_n-D  NumberOfTableDimensions=1  BreakpointsForDimension1=t_d(1,:)  BreakpointsForDimension2=t_d(1,:)  Table=Q_d((r-1)*2+2,:)  InternalRulePriority=Speed  RndMeth=Simplest  InputSameDT=on
  Q_r,d : Outport
  wires:
  t/1 -> Q_r,d,y/1, Q_r,d,x/1
  Q_r,d,y/1 -> Mux/2
  Q_r,d,x/1 -> Mux/1
  Mux/1 -> Q_r,d/1

== system iff_sim/High-authority control/CTC/inverse kinematics/t -> qtt_d/rod 5 ==
  t : Inport
  Mux : Mux  Inputs=2
  Q_r,d,x : Lookup_n-D  NumberOfTableDimensions=1  BreakpointsForDimension1=t_d(1,:)  BreakpointsForDimension2=t_d(1,:)  Table=Q_d((r-1)*2+1,:)  InternalRulePriority=Speed  RndMeth=Simplest  InputSameDT=on
  Q_r,d,y : Lookup_n-D  NumberOfTableDimensions=1  BreakpointsForDimension1=t_d(1,:)  BreakpointsForDimension2=t_d(1,:)  Table=Q_d((r-1)*2+2,:)  InternalRulePriority=Speed  RndMeth=Simplest  InputSameDT=on
  Q_r,d : Outport
  wires:
  t/1 -> Q_r,d,y/1, Q_r,d,x/1
  Q_r,d,y/1 -> Mux/2
  Q_r,d,x/1 -> Mux/1
  Mux/1 -> Q_r,d/1

== system iff_sim/High-authority control/CTC/inverse kinematics/t -> qtt_d/rod 6 ==
  t : Inport
  Mux : Mux  Inputs=2
  Q_r,d,x : Lookup_n-D  NumberOfTableDimensions=1  BreakpointsForDimension1=t_d(1,:)  BreakpointsForDimension2=t_d(1,:)  Table=Q_d((r-1)*2+1,:)  InternalRulePriority=Speed  RndMeth=Simplest  InputSameDT=on
  Q_r,d,y : Lookup_n-D  NumberOfTableDimensions=1  BreakpointsForDimension1=t_d(1,:)  BreakpointsForDimension2=t_d(1,:)  Table=Q_d((r-1)*2+2,:)  InternalRulePriority=Speed  RndMeth=Simplest  InputSameDT=on
  Q_r,d : Outport
  wires:
  t/1 -> Q_r,d,y/1, Q_r,d,x/1
  Q_r,d,y/1 -> Mux/2
  Q_r,d,x/1 -> Mux/1
  Mux/1 -> Q_r,d/1

== system iff_sim/High-authority control/CTC/inverse kinematics/t -> qtt_d/upper base ==
  t : Inport
  Mux : Mux  Inputs=6
  Q_ub,d,phi_x : Lookup_n-D  NumberOfTableDimensions=1  BreakpointsForDimension1=t_d(1,:)  BreakpointsForDimension2=t_d(1,:)  Table=Q_d(16,:)  InternalRulePriority=Speed  RndMeth=Simplest  InputSameDT=on
  Q_ub,d,phi_y : Lookup_n-D  NumberOfTableDimensions=1  BreakpointsForDimension1=t_d(1,:)  BreakpointsForDimension2=t_d(1,:)  Table=Q_d(17,:)  InternalRulePriority=Speed  RndMeth=Simplest  InputSameDT=on
  Q_ub,d,phi_z : Lookup_n-D  NumberOfTableDimensions=1  BreakpointsForDimension1=t_d(1,:)  BreakpointsForDimension2=t_d(1,:)  Table=Q_d(18,:)  InternalRulePriority=Speed  RndMeth=Simplest  InputSameDT=on
  Q_ub,d,x : Lookup_n-D  NumberOfTableDimensions=1  BreakpointsForDimension1=t_d(1,:)  BreakpointsForDimension2=t_d(1,:)  Table=Q_d(13,:)  InternalRulePriority=Speed  RndMeth=Simplest  InputSameDT=on
  Q_ub,d,y : Lookup_n-D  NumberOfTableDimensions=1  BreakpointsForDimension1=t_d(1,:)  BreakpointsForDimension2=t_d(1,:)  Table=Q_d(14,:)  InternalRulePriority=Speed  RndMeth=Simplest  InputSameDT=on
  Q_ub,d,z : Lookup_n-D  NumberOfTableDimensions=1  BreakpointsForDimension1=t_d(1,:)  BreakpointsForDimension2=t_d(1,:)  Table=Q_d(15,:)  InternalRulePriority=Speed  RndMeth=Simplest  InputSameDT=on
  Q_ub,d : Outport
  wires:
  t/1 -> Q_ub,d,y/1, Q_ub,d,z/1, Q_ub,d,phi_x/1, Q_ub,d,phi_y/1, Q_ub,d,phi_z/1, Q_ub,d,x/1
  Q_ub,d,x/1 -> Mux/1
  Q_ub,d,phi_z/1 -> Mux/6
  Q_ub,d,phi_y/1 -> Mux/5
  Q_ub,d,phi_x/1 -> Mux/4
  Q_ub,d,z/1 -> Mux/3
  Q_ub,d,y/1 -> Mux/2
  Mux/1 -> Q_ub,d/1

== system iff_sim/High-authority control/CTC/computed torque control/bases + rods/lower base/O_lb -> G_1 ==
  rot z : sm_lib/Frames and Transforms/Rigid Transform  TranslationMethod=None  TranslationStandardOffset=0  TranslationLengthUnit=m  TranslationStandardAxis=+Z  TranslationCartesianOffset=[0 0 0]  TranslationROffset=0  TranslationROffsetUnits=m  TranslationZOffset=0  TranslationZOffsetUnits=m  TranslationThetaOffset=0  TranslationThetaOffsetUnits=deg  RotationMethod=StandardAxis  RotationAngleUnits=rad  RotationStandardAxis=+Z  RotationAngle=Fi_b_z(1)  RotationArbitraryAxis=[0 0 1]  FollAlignAxisA=+X  BaseAlignAxisA=+Y  FollAlignAxisB=+Y  BaseAlignAxisB=+Z  RotationSequenceAxes=FollowerAxes  RotationSequence=XYX  RotationSequenceAngles=[0 0 0]  RotationSequenceAnglesUnits=deg  RotationMatrix=[1 0 0; 0 1 0; 0 0 1]
  trans z : sm_lib/Frames and Transforms/Rigid Transform  TranslationMethod=StandardAxis  TranslationStandardOffset=h_lb  TranslationLengthUnit=m  TranslationStandardAxis=+Z  TranslationCartesianOffset=[0 0 0]  TranslationROffset=0  TranslationROffsetUnits=m  TranslationZOffset=0  TranslationZOffsetUnits=m  TranslationThetaOffset=0  TranslationThetaOffsetUnits=deg  RotationMethod=None  RotationAngleUnits=deg  RotationStandardAxis=+Z  RotationAngle=0.0  RotationArbitraryAxis=[0 0 1]  FollAlignAxisA=+X  BaseAlignAxisA=+Y  FollAlignAxisB=+Y  BaseAlignAxisB=+Z  RotationSequenceAxes=FollowerAxes  RotationSequence=XYX  RotationSequenceAngles=[0 0 0]  RotationSequenceAnglesUnits=deg  RotationMatrix=[1 0 0; 0 1 0; 0 0 1]
  transl y : sm_lib/Frames and Transforms/Rigid Transform  TranslationMethod=StandardAxis  TranslationStandardOffset=w_lb/2  TranslationLengthUnit=m  TranslationStandardAxis=+Y  TranslationCartesianOffset=[0 0 0]  TranslationROffset=0  TranslationROffsetUnits=m  TranslationZOffset=0  TranslationZOffsetUnits=m  TranslationThetaOffset=0  TranslationThetaOffsetUnits=deg  RotationMethod=None  RotationAngleUnits=deg  RotationStandardAxis=+Z  RotationAngle=0.0  RotationArbitraryAxis=[0 0 1]  FollAlignAxisA=+X  BaseAlignAxisA=+Y  FollAlignAxisB=+Y  BaseAlignAxisB=+Z  RotationSequenceAxes=FollowerAxes  RotationSequence=XYX  RotationSequenceAngles=[0 0 0]  RotationSequenceAnglesUnits=deg  RotationMatrix=[1 0 0; 0 1 0; 0 0 1]
  O_lb : PMIOPort  Side=Left
  G_1 : PMIOPort  Port=2  Side=Right
  connections:
  trans z/LConn1 -- O_lb/RConn1
  trans z/RConn1 -- rot z/LConn1
  transl y/LConn1 -- rot z/RConn1
  transl y/RConn1 -- G_1/RConn1

== system iff_sim/High-authority control/CTC/computed torque control/bases + rods/lower base/O_lb -> G_2 ==
  rot z : sm_lib/Frames and Transforms/Rigid Transform  TranslationMethod=None  TranslationStandardOffset=0  TranslationLengthUnit=m  TranslationStandardAxis=+Z  TranslationCartesianOffset=[0 0 0]  TranslationROffset=0  TranslationROffsetUnits=m  TranslationZOffset=0  TranslationZOffsetUnits=m  TranslationThetaOffset=0  TranslationThetaOffsetUnits=deg  RotationMethod=StandardAxis  RotationAngleUnits=rad  RotationStandardAxis=+Z  RotationAngle=Fi_b_z(2)  RotationArbitraryAxis=[0 0 1]  FollAlignAxisA=+X  BaseAlignAxisA=+Y  FollAlignAxisB=+Y  BaseAlignAxisB=+Z  RotationSequenceAxes=FollowerAxes  RotationSequence=XYX  RotationSequenceAngles=[0 0 0]  RotationSequenceAnglesUnits=deg  RotationMatrix=[1 0 0; 0 1 0; 0 0 1]
  trans z : sm_lib/Frames and Transforms/Rigid Transform  TranslationMethod=StandardAxis  TranslationStandardOffset=h_lb  TranslationLengthUnit=m  TranslationStandardAxis=+Z  TranslationCartesianOffset=[0 0 0]  TranslationROffset=0  TranslationROffsetUnits=m  TranslationZOffset=0  TranslationZOffsetUnits=m  TranslationThetaOffset=0  TranslationThetaOffsetUnits=deg  RotationMethod=None  RotationAngleUnits=deg  RotationStandardAxis=+Z  RotationAngle=0.0  RotationArbitraryAxis=[0 0 1]  FollAlignAxisA=+X  BaseAlignAxisA=+Y  FollAlignAxisB=+Y  BaseAlignAxisB=+Z  RotationSequenceAxes=FollowerAxes  RotationSequence=XYX  RotationSequenceAngles=[0 0 0]  RotationSequenceAnglesUnits=deg  RotationMatrix=[1 0 0; 0 1 0; 0 0 1]
  transl y : sm_lib/Frames and Transforms/Rigid Transform  TranslationMethod=StandardAxis  TranslationStandardOffset=w_lb/2  TranslationLengthUnit=m  TranslationStandardAxis=+Y  TranslationCartesianOffset=[0 0 0]  TranslationROffset=0  TranslationROffsetUnits=m  TranslationZOffset=0  TranslationZOffsetUnits=m  TranslationThetaOffset=0  TranslationThetaOffsetUnits=deg  RotationMethod=None  RotationAngleUnits=deg  RotationStandardAxis=+Z  RotationAngle=0.0  RotationArbitraryAxis=[0 0 1]  FollAlignAxisA=+X  BaseAlignAxisA=+Y  FollAlignAxisB=+Y  BaseAlignAxisB=+Z  RotationSequenceAxes=FollowerAxes  RotationSequence=XYX  RotationSequenceAngles=[0 0 0]  RotationSequenceAnglesUnits=deg  RotationMatrix=[1 0 0; 0 1 0; 0 0 1]
  O_lb : PMIOPort  Side=Left
  G_1 : PMIOPort  Port=2  Side=Right
  connections:
  trans z/LConn1 -- O_lb/RConn1
  trans z/RConn1 -- rot z/LConn1
  transl y/LConn1 -- rot z/RConn1
  transl y/RConn1 -- G_1/RConn1

== system iff_sim/High-authority control/CTC/computed torque control/bases + rods/lower base/O_lb -> G_3 ==
  rot z : sm_lib/Frames and Transforms/Rigid Transform  TranslationMethod=None  TranslationStandardOffset=0  TranslationLengthUnit=m  TranslationStandardAxis=+Z  TranslationCartesianOffset=[0 0 0]  TranslationROffset=0  TranslationROffsetUnits=m  TranslationZOffset=0  TranslationZOffsetUnits=m  TranslationThetaOffset=0  TranslationThetaOffsetUnits=deg  RotationMethod=StandardAxis  RotationAngleUnits=rad  RotationStandardAxis=+Z  RotationAngle=Fi_b_z(3)  RotationArbitraryAxis=[0 0 1]  FollAlignAxisA=+X  BaseAlignAxisA=+Y  FollAlignAxisB=+Y  BaseAlignAxisB=+Z  RotationSequenceAxes=FollowerAxes  RotationSequence=XYX  RotationSequenceAngles=[0 0 0]  RotationSequenceAnglesUnits=deg  RotationMatrix=[1 0 0; 0 1 0; 0 0 1]
  trans z : sm_lib/Frames and Transforms/Rigid Transform  TranslationMethod=StandardAxis  TranslationStandardOffset=h_lb  TranslationLengthUnit=m  TranslationStandardAxis=+Z  TranslationCartesianOffset=[0 0 0]  TranslationROffset=0  TranslationROffsetUnits=m  TranslationZOffset=0  TranslationZOffsetUnits=m  TranslationThetaOffset=0  TranslationThetaOffsetUnits=deg  RotationMethod=None  RotationAngleUnits=deg  RotationStandardAxis=+Z  RotationAngle=0.0  RotationArbitraryAxis=[0 0 1]  FollAlignAxisA=+X  BaseAlignAxisA=+Y  FollAlignAxisB=+Y  BaseAlignAxisB=+Z  RotationSequenceAxes=FollowerAxes  RotationSequence=XYX  RotationSequenceAngles=[0 0 0]  RotationSequenceAnglesUnits=deg  RotationMatrix=[1 0 0; 0 1 0; 0 0 1]
  transl y : sm_lib/Frames and Transforms/Rigid Transform  TranslationMethod=StandardAxis  TranslationStandardOffset=w_lb/2  TranslationLengthUnit=m  TranslationStandardAxis=+Y  TranslationCartesianOffset=[0 0 0]  TranslationROffset=0  TranslationROffsetUnits=m  TranslationZOffset=0  TranslationZOffsetUnits=m  TranslationThetaOffset=0  TranslationThetaOffsetUnits=deg  RotationMethod=None  RotationAngleUnits=deg  RotationStandardAxis=+Z  RotationAngle=0.0  RotationArbitraryAxis=[0 0 1]  FollAlignAxisA=+X  BaseAlignAxisA=+Y  FollAlignAxisB=+Y  BaseAlignAxisB=+Z  RotationSequenceAxes=FollowerAxes  RotationSequence=XYX  RotationSequenceAngles=[0 0 0]  RotationSequenceAnglesUnits=deg  RotationMatrix=[1 0 0; 0 1 0; 0 0 1]
  O_lb : PMIOPort  Side=Left
  G_1 : PMIOPort  Port=2  Side=Right
  connections:
  trans z/LConn1 -- O_lb/RConn1
  trans z/RConn1 -- rot z/LConn1
  transl y/LConn1 -- rot z/RConn1
  transl y/RConn1 -- G_1/RConn1

== system iff_sim/High-authority control/CTC/computed torque control/bases + rods/lower base/wf -> O_lb ==
  rot x : sm_lib/Frames and Transforms/Rigid Transform  TranslationMethod=None  TranslationStandardOffset=0  TranslationLengthUnit=m  TranslationStandardAxis=+Z  TranslationCartesianOffset=[0 0 0]  TranslationROffset=0  TranslationROffsetUnits=m  TranslationZOffset=0  TranslationZOffsetUnits=m  TranslationThetaOffset=0  TranslationThetaOffsetUnits=deg  RotationMethod=StandardAxis  RotationAngleUnits=rad  RotationStandardAxis=+X  RotationAngle=O_lb(4,1)  RotationArbitraryAxis=[0 0 1]  FollAlignAxisA=+X  BaseAlignAxisA=+Y  FollAlignAxisB=+Y  BaseAlignAxisB=+Z  RotationSequenceAxes=FollowerAxes  RotationSequence=XYX  RotationSequenceAngles=[0 0 0]  RotationSequenceAnglesUnits=deg  RotationMatrix=[1 0 0; 0 1 0; 0 0 1]
  rot y : sm_lib/Frames and Transforms/Rigid Transform  TranslationMethod=None  TranslationStandardOffset=0  TranslationLengthUnit=m  TranslationStandardAxis=+Z  TranslationCartesianOffset=[0 0 0]  TranslationROffset=0  TranslationROffsetUnits=m  TranslationZOffset=0  TranslationZOffsetUnits=m  TranslationThetaOffset=0  TranslationThetaOffsetUnits=deg  RotationMethod=StandardAxis  RotationAngleUnits=rad  RotationStandardAxis=+Y  RotationAngle=O_lb(5,1)  RotationArbitraryAxis=[0 0 1]  FollAlignAxisA=+X  BaseAlignAxisA=+Y  FollAlignAxisB=+Y  BaseAlignAxisB=+Z  RotationSequenceAxes=FollowerAxes  RotationSequence=XYX  RotationSequenceAngles=[0 0 0]  RotationSequenceAnglesUnits=deg  RotationMatrix=[1 0 0; 0 1 0; 0 0 1]
  rot z : sm_lib/Frames and Transforms/Rigid Transform  TranslationMethod=None  TranslationStandardOffset=0  TranslationLengthUnit=m  TranslationStandardAxis=+Z  TranslationCartesianOffset=[0 0 0]  TranslationROffset=0  TranslationROffsetUnits=m  TranslationZOffset=0  TranslationZOffsetUnits=m  TranslationThetaOffset=0  TranslationThetaOffsetUnits=deg  RotationMethod=StandardAxis  RotationAngleUnits=rad  RotationStandardAxis=+X  RotationAngle=O_lb(6,1)  RotationArbitraryAxis=[0 0 1]  FollAlignAxisA=+X  BaseAlignAxisA=+Y  FollAlignAxisB=+Y  BaseAlignAxisB=+Z  RotationSequenceAxes=FollowerAxes  RotationSequence=XYX  RotationSequenceAngles=[0 0 0]  RotationSequenceAnglesUnits=deg  RotationMatrix=[1 0 0; 0 1 0; 0 0 1]
  transl : sm_lib/Frames and Transforms/Rigid Transform  TranslationMethod=Cartesian  TranslationStandardOffset=0  TranslationLengthUnit=m  TranslationStandardAxis=+Z  TranslationCartesianOffset=O_lb(1:3,1)  TranslationROffset=0  TranslationROffsetUnits=m  TranslationZOffset=0  TranslationZOffsetUnits=m  TranslationThetaOffset=0  TranslationThetaOffsetUnits=deg  RotationMethod=None  RotationAngleUnits=deg  RotationStandardAxis=+Z  RotationAngle=0.0  RotationArbitraryAxis=[0 0 1]  FollAlignAxisA=+X  BaseAlignAxisA=+Y  FollAlignAxisB=+Y  BaseAlignAxisB=+Z  RotationSequenceAxes=FollowerAxes  RotationSequence=XYX  RotationSequenceAngles=[0 0 0]  RotationSequenceAnglesUnits=deg  RotationMatrix=[1 0 0; 0 1 0; 0 0 1]
  wf : PMIOPort  Side=Left
  O_lb : PMIOPort  Port=2  Side=Right
  connections:
  transl/LConn1 -- wf/RConn1
  transl/RConn1 -- rot x/LConn1
  rot x/RConn1 -- rot y/LConn1
  rot y/RConn1 -- rot z/LConn1
  O_lb/RConn1 -- rot z/RConn1
